simulink model "LateralControlTutorial"  (R2019a)
settings: Solver=FixedStepAuto  StartTime=0.0  StopTime=simStopTime  FixedStep=1e-3  MaxStep=1e-2  MinStep=1e-3  RelTol=5e-3
PostLoadFcn:
  | addpath(fullfile(matlabroot,'toolbox','shared','drivingscenario'));
  | helperLateralControlTutorialSetup
values from neighbouring files (symbols this model uses):
  directions = obj.DirectionsInternal    [HelperPathAnalyzer.m]
  refPoses = driving.internal.control.rearPoseToFrontPose(refPoses, obj.Wheelbase)    [HelperPathAnalyzer.m]
  wheelbase = obj.Wheelbase    [HelperPathAnalyzer.m]
undefined symbols (not defined in the file or in its folder): curvatures, speed, speedProfile, theta0, x0, y0
libraries: drivingvehiclecontroller x2, autolibshared x1, simulink_extras x1, drivingscenarioandsensors x1
settings Model: PacingRate=0.750000  Creator=The MathWorks, Inc.  LastModifiedBy=The MathWorks, Inc.
settings SolverCC: ZeroCrossAlgorithm=Adaptive  DecoupledContinuousIntegration=on  MinimalZcImpactIntegration=on
settings DataIOCC: SaveOutput=off  SignalLogging=off  DSMLogging=off  SaveTime=off  ReturnWorkspaceOutputs=off
settings DebuggingCC: PregeneratedLibrarySubsystemCodeDiagnostic=none  ArithmeticOperatorsInVariantConditions=warning
settings SFSimCC: SimUseLocalCustomCode=off
settings RTWCC: RTWUseLocalCustomCode=off

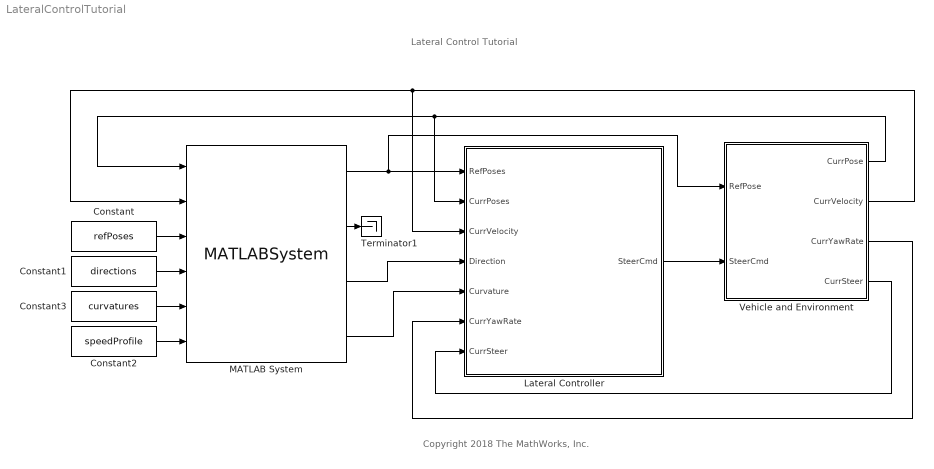
== system LateralControlTutorial ==
  note: Lateral Control Tutorial
  note: Copyright 2018 The MathWorks, Inc.
  Constant : Constant  Value=refPoses
  Constant1 : Constant  Value=directions
  Constant2 : Constant  Value=speedProfile
  Constant3 : Constant  Value=curvatures
  Lateral Controller : Subsystem  VariantControlMode=Label  Variant=on  VariantControl=Kinematic  LabelModeActiveChoice=Kinematic
  MATLAB System : MATLABSystem  System=HelperPathAnalyzer  Wheelbase=wheelbase  HasResetOutput=off  SimulateUsing=Interpreted execution
      mask Type: HelperPathAnalyzer
      mask Display:
      | disp(['Helper' char(10) 'Path' char(10) 'Analyzer']);
      | port_label('input',1,'CurrPose');
      | port_label('input',2,'CurrVelocity');
      | port_label('input',3,'RefPoses');
      | port_label('input',4,'Directions');
      | port_label('input',5,'Curvatures');
      | port_label('input',6,'SpeedProfile');
      | port_label('output',1,'RefPose');
      | port_label('output',2,'RefVelocity');
      | port_label('output',3,'Direction');
      | port_label('output',4,'Curvature');
  Terminator1 : Terminator
  Vehicle and Environment : Subsystem
  wires:
  Constant/1 -> MATLAB System/3
  MATLAB System/2 -> Terminator1/1
  Constant1/1 -> MATLAB System/4
  Vehicle and Environment/1(CurrPose) -> MATLAB System/1, Lateral Controller/2("CurrPoses ")
  Vehicle and Environment/2(CurrVelocity) -> MATLAB System/2, Lateral Controller/3("CurrVelocity ")
  MATLAB System/1 -> Lateral Controller/1("RefPoses "), Vehicle and Environment/1(RefPose)
  MATLAB System/3 -> Lateral Controller/4("Direction ")
  MATLAB System/4 -> Lateral Controller/5("Curvature ")
  Lateral Controller/1(" SteerCmd") -> Vehicle and Environment/2(SteerCmd)
  Vehicle and Environment/4(CurrSteer) -> Lateral Controller/7("CurrSteer ")
  Vehicle and Environment/3(CurrYawRate) -> Lateral Controller/6("CurrYawRate ")
  Constant2/1 -> MATLAB System/6
  Constant3/1 -> MATLAB System/5

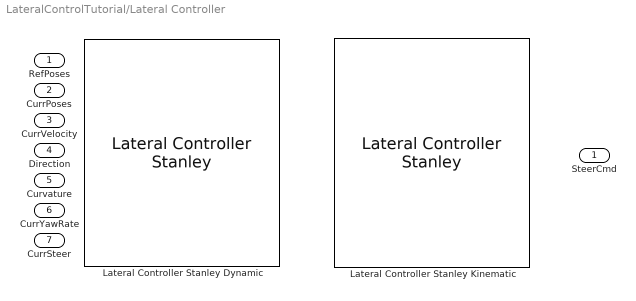
== system LateralControlTutorial/Lateral Controller ==
  "RefPoses " : Inport
  "CurrPoses " : Inport  Port=2
  "CurrVelocity " : Inport  Port=3
  "Direction " : Inport  Port=4
  "Curvature " : Inport  Port=5
  "CurrYawRate " : Inport  Port=6
  "CurrSteer " : Inport  Port=7
  Lateral Controller Stanley Dynamic : drivingvehiclecontroller/Lateral Controller Stanley  VariantControl=Dynamic  ModelType=Dynamic bicycle model  PositionGainF=2  PositionGainR=2.5  YawRateGain=0.5  DelayGain=0.2  VehicleMass=1575  Lf=1.2  Lr=1.6  TireStiffness=19000  Wheelbase=wheelbase  MaxSteeringAngle=35
      settings: SourceProductName=Automated Driving Toolbox  SourceProductBaseCode=DR
  Lateral Controller Stanley Kinematic : drivingvehiclecontroller/Lateral Controller Stanley  VariantControl=Kinematic  ModelType=Kinematic bicycle model  PositionGainF=2  PositionGainR=2.5  YawRateGain=0.2  DelayGain=0.2  VehicleMass=1575  Lf=1.2  Lr=1.6  TireStiffness=19000  Wheelbase=wheelbase  MaxSteeringAngle=35
      settings: SourceProductName=Automated Driving Toolbox  SourceProductBaseCode=DR
  " SteerCmd" : Outport

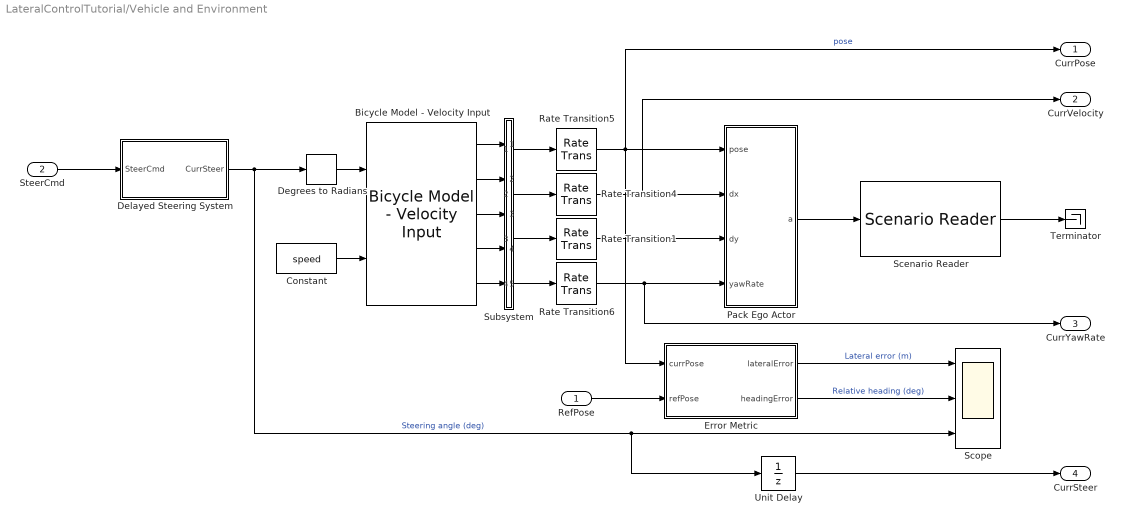
== system LateralControlTutorial/Vehicle and Environment ==
  RefPose : Inport
  SteerCmd : Inport  Port=2
  Bicycle Model - Velocity Input : autolibshared/Bicycle Model - Velocity Input  trackMode=Single (bicycle)  inputMode=External longitudinal forces  frontSteerMode=on  rearSteerMode=off  windMode=off  muMode=off  extFMode=off  extMMode=off  aMode=3  NF=2  NR=2  m=1575  a=1.2  b=1.6  h=0.35  X_o=x0+cosd(theta0)*1.6  xdot_o=0  CalphaMode=off  sigmaMode=on  w=[1.4,1.4]  Cy_f=19e3  Cy_r=20e3  sigma_f=.1  sigma_r=.1  alpha_f_brk=[-.1 .1]  Cy_f_data=[-9e3 9e3]  alpha_r_brk=[-.1 .1]  Cy_r_data=[-9e3 9e3]  Y_o=y0+sind(theta0)*1.6  ydot_o=0  Izz=4000  psi_o=deg2rad(theta0)  r_o=0  Af=2  Cd=.3  Cl=.1  Cpm=.1  beta_w=[0:0.01:0.3]  Cs=[0:0.03:0.9]  Cym=[0:0.01:0.3]  Pabs=101325  Tair=273  g=9.81  mu=1  xdot_tol=.01  Fznom=5000  Fxtire_sat=1e6  Fytire_sat=1e6  longOff=0  latOff=0  vertOff=0
      settings: SourceProductName=Powertrain Blockset  SourceProductBaseCode=PW
  Constant : Constant  Value=speed
  Degrees to Radians : simulink_extras/Transformations/Degrees to Radians
  Delayed Steering System : Subsystem
  Error Metric : MATLAB Function  TreatAsAtomicUnit=on  mask{wheelbase=wheelbase}
      mask prompts: wheelbase "Wheelbase of vehicle"
  Pack Ego Actor : MATLAB Function  TreatAsAtomicUnit=on
  Rate Transition1 : RateTransition  OutPortSampleTime=Ts
  Rate Transition4 : RateTransition  InitialCondition=speed  OutPortSampleTime=Ts
  Rate Transition5 : RateTransition  InitialCondition=[x0, y0, theta0]  OutPortSampleTime=Ts
  Rate Transition6 : RateTransition  OutPortSampleTime=Ts
  Scenario Reader : drivingscenarioandsensors/Scenario Reader  ScenarioFileName=LateralControl.mat  OutputCoordinateSystem=Vehicle coordinates  EgoVehicleSource=Input port  SampleTime=0.05  LaneBoundaryOutput=None  LaneBoundaryDistance=0:0.5:9.5  LaneBoundaryLocation=Center of lane markings  BusNameSource=Auto  BusName2Source=Auto  SimulateUsing=Interpreted execution
      settings: SourceProductName=Automated Driving Toolbox
  Scope : Scope  NumInputPorts=3
  Subsystem : Subsystem
  Terminator : Terminator
  Unit Delay : UnitDelay  SampleTime=0.05  HasFrameUpgradeWarning=on
  CurrPose : Outport
  CurrVelocity : Outport  Port=2
  CurrYawRate : Outport  Port=3
  CurrSteer : Outport  Port=4
  wires:
  Rate Transition4/1 -> Pack Ego Actor/2(dx), CurrVelocity/1
  Subsystem/3(Out3) -> Rate Transition1/1
  Subsystem/2(Out2) -> Rate Transition4/1
  Subsystem/1(Out1) -> Rate Transition5/1
  Rate Transition6/1 -> CurrYawRate/1, Pack Ego Actor/4(yawRate)
  Subsystem/4(Out4) -> Rate Transition6/1
  Rate Transition1/1 -> Pack Ego Actor/3(dy)
  Rate Transition5/1 -> Error Metric/1(currPose), Pack Ego Actor/1(pose), CurrPose/1  "pose"
  Error Metric/1(lateralError) -> Scope/1  "Lateral error (m)"
  RefPose/1 -> Error Metric/2(refPose)
  SteerCmd/1 -> Delayed Steering System/1(SteerCmd)
  Error Metric/2(headingError) -> Scope/2  "Relative heading (deg)"
  Degrees to Radians/1 -> Bicycle Model - Velocity Input/1
  Constant/1 -> Bicycle Model - Velocity Input/2
  Bicycle Model - Velocity Input/4 -> Subsystem/4(In4)
  Bicycle Model - Velocity Input/5 -> Subsystem/5(In5)
  Bicycle Model - Velocity Input/1 -> Subsystem/1(In1)
  Bicycle Model - Velocity Input/2 -> Subsystem/2(In2)
  Bicycle Model - Velocity Input/3 -> Subsystem/3(In3)
  Delayed Steering System/1(CurrSteer) -> Degrees to Radians/1, Unit Delay/1, Scope/3  "Steering angle (deg)"
  Unit Delay/1 -> CurrSteer/1
  Pack Ego Actor/1(a) -> Scenario Reader/1
  Scenario Reader/1 -> Terminator/1

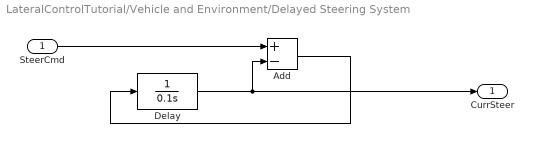
== system LateralControlTutorial/Vehicle and Environment/Delayed Steering System ==
  SteerCmd : Inport
  Add : Sum  Inputs=+-
  Delay : TransferFcn  Denominator=[0.1 0]
  CurrSteer : Outport
  wires:
  Add/1 -> Delay/1
  SteerCmd/1 -> Add/1
  Delay/1 -> CurrSteer/1, Add/2

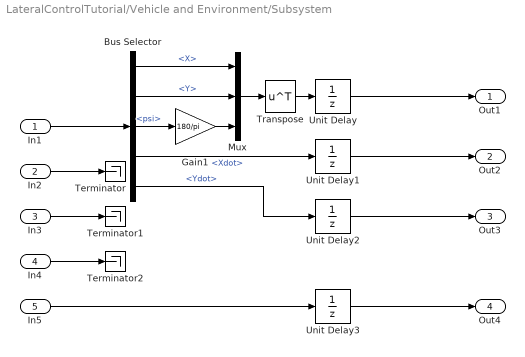
== system LateralControlTutorial/Vehicle and Environment/Subsystem ==
  In1 : Inport
  In2 : Inport  Port=2
  In3 : Inport  Port=3
  In4 : Inport  Port=4
  In5 : Inport  Port=5
  Bus Selector : BusSelector  OutputSignals=InertFrm.RearAxl.Disp.X,InertFrm.RearAxl.Disp.Y,InertFrm.Cg.Ang.psi,InertFrm.RearAxl.Vel.Xdot,InertFrm.RearAxl.Vel.Ydot
  Gain1 : Gain  Gain=180/pi
  Mux : Mux  Inputs=3
  Terminator : Terminator
  Terminator1 : Terminator
  Terminator2 : Terminator
  Transpose : Math  Operator=transpose  SaturateOnIntegerOverflow=on
  Unit Delay : UnitDelay  InitialCondition=[x0, y0, theta0]  SampleTime=-1  HasFrameUpgradeWarning=on
  Unit Delay1 : UnitDelay  InitialCondition=speed  SampleTime=-1  HasFrameUpgradeWarning=on
  Unit Delay2 : UnitDelay  SampleTime=-1  HasFrameUpgradeWarning=on
  Unit Delay3 : UnitDelay  SampleTime=-1  HasFrameUpgradeWarning=on
  Out1 : Outport
  Out2 : Outport  Port=2
  Out3 : Outport  Port=3
  Out4 : Outport  Port=4
  wires:
  Bus Selector/4 -> Unit Delay1/1  "<Xdot>"
  Bus Selector/2 -> Mux/2  "<Y>"
  Bus Selector/1 -> Mux/1  "<X>"
  Transpose/1 -> Unit Delay/1
  Unit Delay/1 -> Out1/1
  Mux/1 -> Transpose/1
  Unit Delay3/1 -> Out4/1
  Bus Selector/5 -> Unit Delay2/1  "<Ydot>"
  Bus Selector/3 -> Gain1/1  "<psi>"
  Gain1/1 -> Mux/3
  In5/1 -> Unit Delay3/1
  In2/1 -> Terminator/1
  In1/1 -> Bus Selector/1
  In4/1 -> Terminator2/1
  Unit Delay2/1 -> Out3/1
  Unit Delay1/1 -> Out2/1
  In3/1 -> Terminator1/1

== matlab function LateralControlTutorial/Vehicle and Environment/Error Metric ==
  data: currPose input size=[1 3]; refPose input size=[1 3]; lateralError output; wheelbase parameter; headingError output
function [lateralError, headingError] = fcn(currPose, refPose, wheelbase)

%   Copyright 2018 The MathWorks, Inc.

currPose(:,3) = deg2rad(currPose(:,3));
refPose(:,3)  = deg2rad(refPose(:,3));

%Convert current pose to front wheel coordinate
currPoseF = coder.nullcopy(zeros(1, 3));

currPoseF = driving.internal.control.rearPoseToFrontPose(currPose, wheelbase);

lateralError = norm(currPoseF(1:2) - refPose(1:2));

headingError = rad2deg(currPose(:, 3) - refPose(:,3));

== matlab function LateralControlTutorial/Vehicle and Environment/Pack Ego Actor ==
  data: pose input; a output Bus: BusActors1Actors size=1; dx input; dy input; yawRate input
function a = packEgo(pose,dx,dy,yawRate)
% Pack ego information into a single ego actor bus
%
% Imoprtant note:
% Output is a bus of type BusActorsActors. This is the same bus used by the
% Scenario Reader to output an individual actor. If you change the
% output bus name of Scenario Reader, change the output bus name here
% as well by clicking on 'Edit Data' in the menu above.

a = struct(...
    'ActorID',1,...
    'Position', [pose(1) pose(2) 0], ...
    'Velocity', [dx dy 0], ...
    'Roll', 0, ...
    'Pitch', 0, ...
    'Yaw', pose(3), ...
    'AngularVelocity', [0 0 yawRate]);
